simulink model "model_ver_notlin"  (R2020b)
settings: Solver=ode45  StartTime=0.0  StopTime=10  MaxStep=0.01  RelTol=1e-3  AbsTol=1e-3  EnableMultiTasking=on
undefined symbols (not defined in the file): alpha_0, params, w_0
settings Model: Creator=Danil  LastModifiedBy=Danil
settings SolverCC: AutoScaleAbsTol=off
settings DataIOCC: LimitDataPoints=on  MaxDataPoints=10000
settings OptimizationCC: LifeSpan=inf
settings DebuggingCC: AllowSymbolicDim=off  SFUnexpectedBacktrackingDiag=warning  SFNoUnconditionalDefaultTransitionDiag=warning  SFExecutionAtInitializationDiag=none  ArithmeticOperatorsInVariantConditions=warning
settings SFSimCC: SimUseLocalCustomCode=off  CustomCodeUndefinedFunction=UseInterfaceOnly
settings RTWCC: RTWUseLocalCustomCode=off
settings CodeAppCC: StateflowObjectComments=on
settings GRTTargetCC: TargetLangStandard=C89/C90 (ANSI)
settings ConfigComp: CovMetricSettings=dw  CovSaveCumulativeToWorkspaceVar=on  CovSaveSingleToWorkspaceVar=on  CovExternalEMLEnable=off  CovSFcnEnable=off
settings SimscapeCC: SimscapeLogType=all  SimscapeLogSimulationStatistics=on  SimscapeLogDataHistory=10000

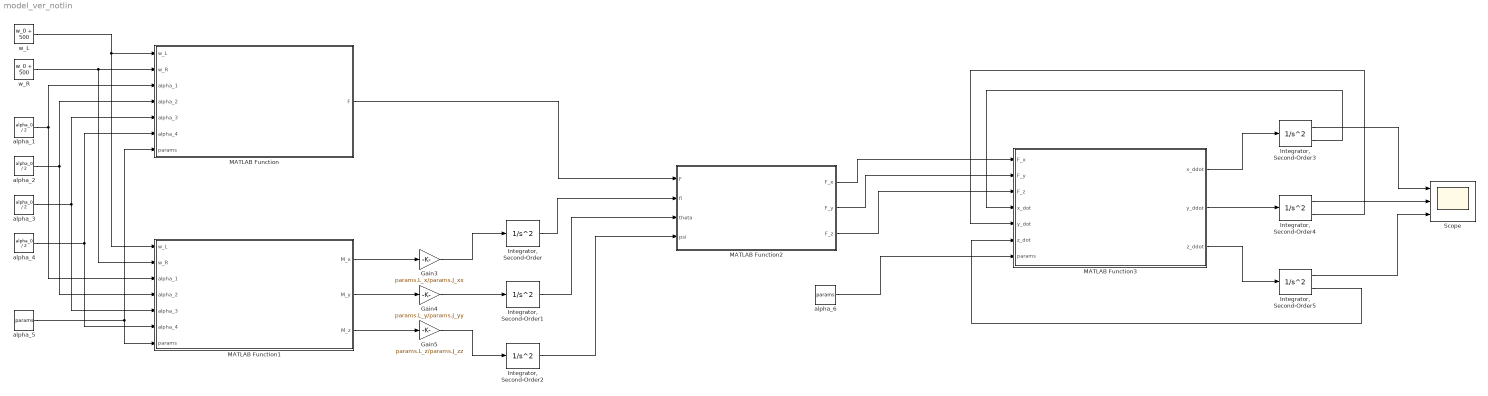
== system model_ver_notlin ==
  Gain3 : Gain  Gain=params.L_x/params.J_xx
  Gain4 : Gain  Gain=params.L_y/params.J_yy
  Gain5 : Gain  Gain=params.L_z/params.J_zz
  "Integrator, Second-Order" : SecondOrderIntegrator  ShowOutput=x
  "Integrator, Second-Order1" : SecondOrderIntegrator  ShowOutput=x
  "Integrator, Second-Order2" : SecondOrderIntegrator  ShowOutput=x
  "Integrator, Second-Order3" : SecondOrderIntegrator
  "Integrator, Second-Order4" : SecondOrderIntegrator
  "Integrator, Second-Order5" : SecondOrderIntegrator
  MATLAB Function : MATLAB Function  TreatAsAtomicUnit=on
  MATLAB Function1 : MATLAB Function  TreatAsAtomicUnit=on
  MATLAB Function2 : MATLAB Function  TreatAsAtomicUnit=on
  MATLAB Function3 : MATLAB Function  TreatAsAtomicUnit=on
  Scope : Scope  NumInputPorts=3
  alpha_{1..4} (4 alike) : Constant  Value=alpha_0 / 2
  alpha_5 : Constant  Value=params  OutDataTypeStr=Bus: params_bus
  alpha_6 : Constant  Value=params  OutDataTypeStr=Bus: params_bus
  w_L : Constant  Value=w_0 + 500
  w_R : Constant  Value=w_0 + 500
  wires:
  MATLAB Function1/2(M_y) -> Gain4/1
  MATLAB Function1/1(M_x) -> Gain3/1
  MATLAB Function1/3(M_z) -> Gain5/1
  Gain4/1 -> "Integrator, Second-Order1"/1
  Gain3/1 -> "Integrator, Second-Order"/1
  Gain5/1 -> "Integrator, Second-Order2"/1
  MATLAB Function/1(F) -> MATLAB Function2/1(F)
  "Integrator, Second-Order"/1 -> MATLAB Function2/2(fi)
  "Integrator, Second-Order1"/1 -> MATLAB Function2/3(theta)
  "Integrator, Second-Order2"/1 -> MATLAB Function2/4(psi)
  MATLAB Function2/1(F_x) -> MATLAB Function3/1(F_x)
  MATLAB Function2/2(F_y) -> MATLAB Function3/2(F_y)
  MATLAB Function2/3(F_z) -> MATLAB Function3/3(F_z)
  alpha_6/1 -> MATLAB Function3/7(params)
  w_L/1 -> MATLAB Function/1(w_L), MATLAB Function1/1(w_L)
  w_R/1 -> MATLAB Function1/2(w_R), MATLAB Function/2(w_R)
  alpha_1/1 -> MATLAB Function/3(alpha_1), MATLAB Function1/3(alpha_1)
  alpha_2/1 -> MATLAB Function/4(alpha_2), MATLAB Function1/4(alpha_2)
  alpha_3/1 -> MATLAB Function/5(alpha_3), MATLAB Function1/5(alpha_3)
  alpha_4/1 -> MATLAB Function/6(alpha_4), MATLAB Function1/6(alpha_4)
  alpha_5/1 -> MATLAB Function/7(params), MATLAB Function1/7(params)
  MATLAB Function3/1(x_ddot) -> "Integrator, Second-Order3"/1
  MATLAB Function3/2(y_ddot) -> "Integrator, Second-Order4"/1
  MATLAB Function3/3(z_ddot) -> "Integrator, Second-Order5"/1
  "Integrator, Second-Order3"/2 -> MATLAB Function3/4(x_dot)
  "Integrator, Second-Order4"/2 -> MATLAB Function3/5(y_dot)
  "Integrator, Second-Order5"/2 -> MATLAB Function3/6(z_dot)
  "Integrator, Second-Order4"/1 -> Scope/2
  "Integrator, Second-Order3"/1 -> Scope/1
  "Integrator, Second-Order5"/1 -> Scope/3

== matlab function model_ver_notlin/MATLAB Function1 ==
  data: w_L input; M_x output; w_R input; alpha_1 input; alpha_2 input; alpha_3 input; alpha_4 input; params input; M_y output; M_z output
function [M_x, M_y, M_z] = fcn(w_L, w_R, alpha_1, alpha_2, alpha_3, alpha_4, params)
alpha_1 = alpha_1 * pi / 180;
alpha_2 = alpha_2 * pi / 180;
alpha_3 = alpha_3 * pi / 180;

M_x = params.k_F * (w_L^2 * cos(alpha_1 - alpha_2) - w_R^2 * cos(alpha_3 - alpha_4));
M_y = params.k_F * (w_L^2 * sin(alpha_1 - alpha_2) + w_R^2 * sin(alpha_3 - alpha_4));
M_z = params.k_F * (w_L^2 * sin(alpha_1 - alpha_2) - w_R^2 * sin(alpha_3 - alpha_4));

== matlab function model_ver_notlin/MATLAB Function ==
  data: w_L input; F output; w_R input; alpha_1 input; alpha_2 input; alpha_3 input; alpha_4 input; params input
function F = fcn(w_L, w_R, alpha_1, alpha_2, alpha_3, alpha_4, params)
alpha_L = alpha_1 + alpha_2;
alpha_R = alpha_3 + alpha_4;

C_Y_L = params.a * alpha_L^2 + params.b * alpha_L + params.c;
C_Y_R = params.a * alpha_R^2 + params.b * alpha_R + params.c;

F = (3/2) * params.rho * params.S_l * (C_Y_L * w_L^2 + C_Y_R * w_R^2);

== matlab function model_ver_notlin/MATLAB Function2 ==
  data: F input; F_x output; fi input; theta input; psi input; F_y output; F_z output
function [F_x, F_y, F_z] = fcn(F, fi, theta, psi)

F_x = F * (cos(psi) * sin(theta) + cos(theta) * sin(fi) * sin(psi));
F_y = F * (sin(psi) * sin(theta) - cos(psi) * cos(theta) * sin(fi));
F_z = F * (cos(fi) * cos(theta));

== matlab function model_ver_notlin/MATLAB Function3 ==
  data: F_x input; x_ddot output; F_y input; F_z input; x_dot input; y_dot input; z_dot input; params input; y_ddot output; z_ddot output
function [x_ddot, y_ddot, z_ddot] = fcn(F_x, F_y, F_z, x_dot, y_dot, z_dot, params)

x_ddot = (1 / params.m) * (F_x - params.k_x * x_dot);
y_ddot = (1 / params.m) * (F_y - params.k_y * y_dot);
z_ddot = (1 / params.m) * (F_z + params.C_y_max * (1 / 2) * params.rho * x_dot^2 * params.S_k - params.k_z * z_dot - params.m * params.g);
